simulink model "testYarpSendText_cpp"  (R2014a)
settings: Solver=FixedStepDiscrete  StartTime=0.0  StopTime=10000  FixedStep=0.002  RelTol=1e-3
model workspace (MAT data in the model file):
  gtest = 0
settings Model: Creator=Ulysses  LastModifiedBy=Ulysses

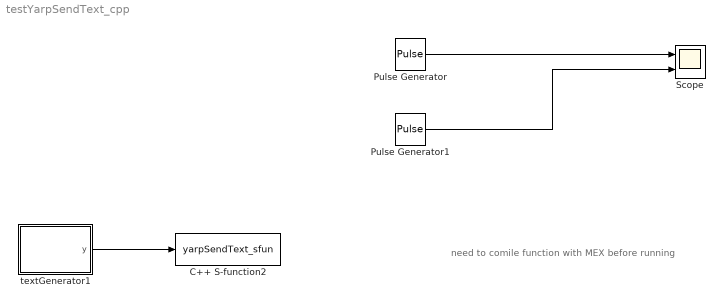
== system testYarpSendText_cpp ==
  note: need to comile function with MEX before running
  C++ S-function2 : S-Function  FunctionName=yarpSendText_sfun  Parameters='/sim/out/smb', '/rs'  EnableBusSupport=off
  Pulse Generator : DiscretePulseGenerator  PulseType=Time based  PulseWidth=5
  Pulse Generator1 : DiscretePulseGenerator  PulseType=Time based  Amplitude=2  PulseWidth=50
  Scope : Scope  NumInputPorts=2
      settings: YMin=-5~-5  YMax=5~5
  textGenerator1 : MATLAB Function  TreatAsAtomicUnit=on
  wires:
  textGenerator1/1(y) -> C++ S-function2/1
  Pulse Generator/1 -> Scope/1
  Pulse Generator1/1 -> Scope/2

== matlab function testYarpSendText_cpp/textGenerator1 ==
  data: y output
function y = fcn()
y = encStr2Arr('test string 2');
